simulink model "test"  (Simulink 7.4)
settings: Solver=ode3  StartTime=0.0  StopTime=22  FixedStep=0.02  RelTol=1e-3
values from neighbouring files (symbols this model uses):
  K = zeros(6,2)    [LQR_code_20190617.m]
undefined symbols (not defined in the file or in its folder): cart, pole, sigbuilder_block, test1
settings Model: Creator=PinkWink  LastModifiedBy=PinkWink

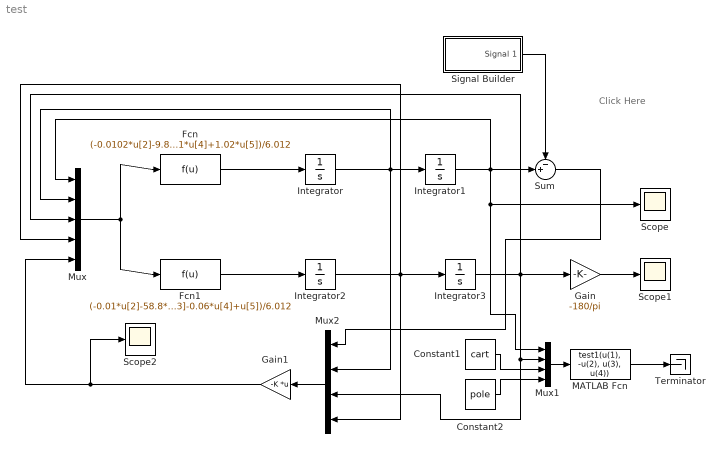
== system test ==
  note: Click Here
  Constant1 : Constant  Value=cart  OutDataType=fixdt(1, 16)  OutScaling=2^0
  Constant2 : Constant  Value=pole  OutDataType=fixdt(1, 16)  OutScaling=2^0
  Fcn : Fcn  Expr=(-0.0102*u[2]-9.8*u[3]-0.01*u[4]+1.02*u[5])/6.012
  Fcn1 : Fcn  Expr=(-0.01*u[2]-58.8*u[3]-0.06*u[4]+u[5])/6.012
  Gain : Gain  Gain=-180/pi  ParameterDataType=fixdt(1, 16)  ParameterScaling=2^0  OutDataType=fixdt(1, 16)  OutScaling=2^0
  Gain1 : Gain  Gain=-K  Multiplication=Matrix(K*u)  ParameterDataType=fixdt(1, 16)  ParameterScaling=2^0  OutDataType=fixdt(1, 16)  OutScaling=2^0
  Integrator{,1..3} (4 alike) : Integrator
  MATLAB Fcn : MATLABFcn  MATLABFcn=test1(u(1), -u(2), u(3), u(4))
  Mux : Mux  Inputs=5
  Mux1 : Mux
  Mux2 : Mux
  Scope : Scope
      settings: YMin=0.72  YMax=0.9
  Scope1 : Scope
  Scope2 : Scope
      settings: YMin=-6  YMax=-4  SaveName=ScopeData2
  Signal Builder : Subsystem  Tag=STV Subsys  LoadFcn=sigbuilder_block('load');  StartFcn=sigbuilder_block('start');  StopFcn=sigbuilder_block('stop');  ClipboardFcn=sigbuilder_block('clipboard');  mask(Sigbuilder block){}
      mask help: Sigbuilder GUI
      mask init:
      | if ~strcmp(get_param(bdroot(gcbh),'SimulationStatus'),'stopped') tuvar = sigbuilder_block('maskInit'); end
      settings: CopyFcn=sigbuilder_block('copy');  DeleteFcn=sigbuilder_block('delete');  ModelCloseFcn=sigbuilder_block('modelClose');  PreSaveFcn=sigbuilder_block('preSave');  NameChangeFcn=sigbuilder_block('namechange');  OpenFcn=sigbuilder_block('open',[429.75 84 548.25 399 ]);  CloseFcn=sigbuilder_block('close');
      mask Display: plot(0,0,100,100,[10,10,40,40,10],[80,20,20,80,80],[40,10],[50,50], [40,27,10],[65,72,56],[40,25,25,10],[28,28,43,43]);
  Sum : Sum  Inputs=-+|  OutDataType=fixdt(1, 16)  OutScaling=2^0
  Terminator : Terminator
  wires:
  Mux/1 -> Fcn/1, Fcn1/1
  Fcn/1 -> Integrator/1
  Integrator/1 -> Integrator1/1, Mux/2, Mux2/2
  Fcn1/1 -> Integrator2/1
  Integrator2/1 -> Integrator3/1, Mux/4, Mux2/4
  Integrator3/1 -> Gain/1, Mux/3, Mux1/2, Mux2/3
  Gain/1 -> Scope1/1
  Mux1/1 -> MATLAB Fcn/1
  MATLAB Fcn/1 -> Terminator/1
  Constant1/1 -> Mux1/3
  Constant2/1 -> Mux1/4
  Mux2/1 -> Gain1/1
  Gain1/1 -> Mux/5, Scope2/1
  Integrator1/1 -> Sum/2, Scope/1, Mux1/1, Mux/1
  Signal Builder/1(Signal 1) -> Sum/1
  Sum/1 -> Mux2/1

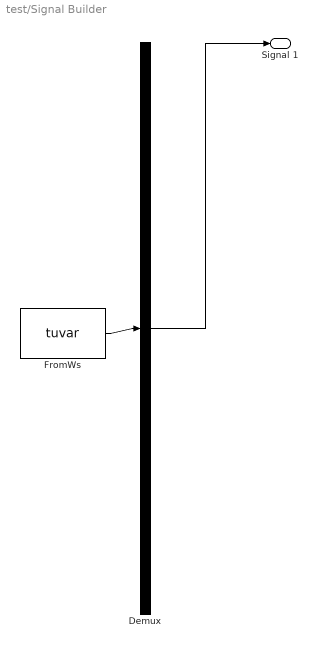
== system test/Signal Builder ==
  Demux : Demux  Tag=STV Demux  Outputs=1
  FromWs : FromWorkspace  Tag=STV FromWs  VariableName=tuvar  SampleTime=0  SigBuilderData=DataTag0  VnvData=DataTag1
      SigBuilderData=|
      | common.afterFinalStr = 'Extrapolate'
      | common.sampleTime = 0
      | dataSet.timeRange = [0 22]
      | dataSet.name = 'Group 1'
      | sbobj.Groups.Name = 'Group 1'
      | sbobj.Groups.Signals.Name = 'Signal 1'
      | sbobj.Groups.Signals.XData = [0 2 2 6 10 10 14 18 20 22]
      | sbobj.Groups.Signals.YData = [0.03 1.99 2 2 -2.04 -2.02 -2 0 0.01 0.01]
  Signal 1 : Outport  Tag=STV Outport  OutDataType=fixdt(1, 16)  OutScaling=2^0
  wires:
  Demux/1 -> Signal 1/1
  FromWs/1 -> Demux/1
